simulink model "Estim_DistCont_Fault_topresent"  (R2018b)
settings: Solver=ode1  StartTime=0.0  StopTime=20000  FixedStep=1  RelTol=1e-3
InitFcn:
  | clearvars
  | addpath('C:\Users\u375749\Documents\Thesis\Codes\Linearization')
  | addpath('C:\Users\u375749\Documents\Thesis\Codes\MatlabPlant')
  | addpath('C:\Users\u375749\Documents\Thesis\Codes\ModelicaPlant\objects_inits')
  | addpath('C:\Users\u375749\Documents\Thesis\Codes\ModelicaPlant\matfiles')
  | addpath('C:\Users\u375749\Documents\Thesis\Codes\ModelicaPlant')
  | modelcreation_simplified
  | substitution_simplified
  | distributedControllers
  | delayT = 300;
  | delayh = 50;% 400*19.2*1e-3*2/0.321;
  | hRatio = 1/3;
  | kfinit_simulink
  | rlsinit_simulink
  | enableFaultOperation = 1;
  | enableBatch = 0;
  | enableTA0fault = 0;
  | faultinit_simulink
  | clear u
values from neighbouring files (symbols this model uses):
  fValues = 48    [faultcontrol3.mat]    (also in faultcontrol4.mat)
  npy = 2    [faultcontrol3.mat]    (also in faultcontrol4.mat)
  nr = 6    [faultcontrol3.mat]    (also in faultcontrol4.mat)
  sigma2p = 277777777.778    [faultcontrol3.mat]    (also in faultcontrol4.mat)
  sigma2T = 0.111111111111    [faultcontrol3.mat]    (also in faultcontrol4.mat)
  sigma2x = 1.11111111111e-05    [faultcontrol3.mat]    (also in faultcontrol4.mat)
  Ts = 1    [faultcontrol3.mat]    (also in faultcontrol4.mat)
  VValues = [0.0192 0.133 0.0001 0.00024]    [faultcontrol3.mat]    (also in faultcontrol4.mat)
undefined symbols (not defined in the file or in its folder): CoolProp, DiscIntNeverNeededParam, fdEM, PI_C, PI_F, PI_GC, PI_HP, PI_LT, PI_MT, PI_RP, rls, x2q
libraries: simulink x6, dspswit3 x1, FMIKit_blocks x1
settings Model: NumberOfSteps=10  Creator=U370698  LastModifiedBy=U375749
settings DebuggingCC: LibraryContextMissingDiagnostic=none  UnderSpecifiedDimensionMsg=warning
settings SFSimCC: SimUseLocalCustomCode=off
settings RTWCC: RTWUseLocalCustomCode=off

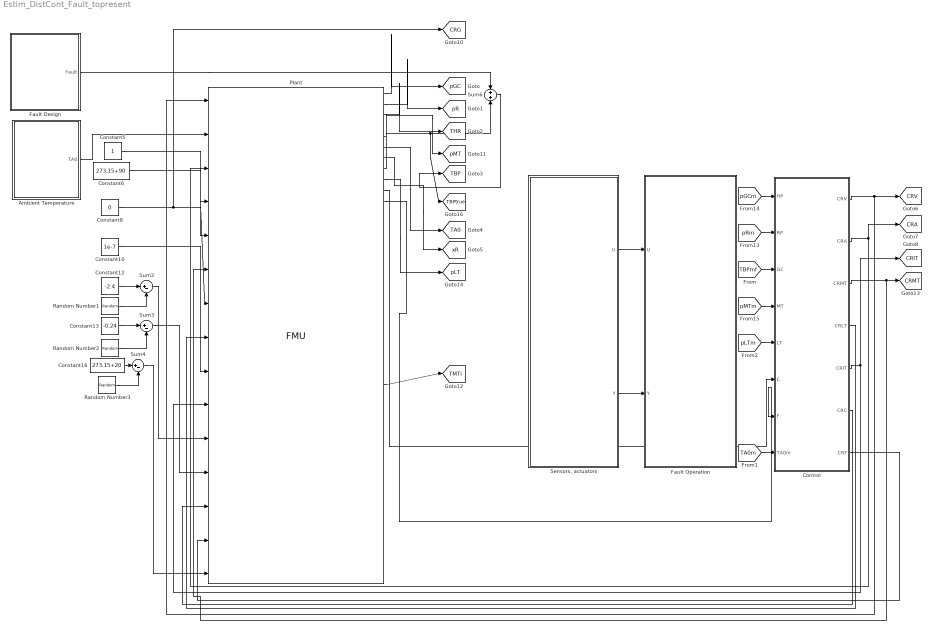
== system Estim_DistCont_Fault_topresent ==
  Ambient Temperature : Subsystem
  Constant10 : Constant  Value=1e-7
  Constant12 : Constant  Value=-2.4
  Constant13 : Constant  Value=-0.24
  Constant16 : Constant  Value=273.15+20
  Constant5 : Constant
  Constant6 : Constant  Value=273.15+90
  Constant8 : Constant  Value=0
  Control : Subsystem
  Fault Design : Subsystem
  Fault Operation : Subsystem
  Plant : FMIKit_blocks/FMU  SFunctionModules=''
      settings: SourceProductName=FMI Kit
  Random Number1 : RandomNumber  Variance=(0.2/3)^2/Ts  Seed=51  SampleTime=1
  Random Number2 : RandomNumber  Variance=(0.02/3)^2/Ts  Seed=52  SampleTime=1
  Random Number3 : RandomNumber  Variance=(1/10)^2/Ts  Seed=53  SampleTime=1
  "Sensors, actuators" : Subsystem
  Sum2 : Sum  Inputs=|+-
  Sum3 : Sum  Inputs=|+-
  Sum4 : Sum  Inputs=|+-
  Sum6 : Sum  Inputs=+|+
  tag scope: CRA=global, CRG=global, CRIT=global, CRMT=global, CRV=global, TA0=global, TBP=global, TBPtrue=global, THR=global, TMTi=global, pGC=global, pLT=global, pMT=global, pR=global, xR=global
  wires:
  Constant5/1 -> Plant/4
  Constant6/1 -> Plant/5
  Constant8/1 -> [CRG], Plant/7
  Constant10/1 -> Plant/9
  Plant/1 -> [pGC]
  Plant/3 -> [THR]
  Control/1(CRV) -> [CRV], Plant/1
  Control/2(CRA) -> [CRA], Plant/3
  Control/3(CRMT) -> Plant/6, [CRMT]
  Control/4(CRLT) -> Plant/8
  Control/6(CRC) -> Plant/13
  Control/7(CRF) -> Plant/14
  Plant/11 -> Control/7(F)
  Plant/10 -> Control/6(C)
  Plant/9 -> [pLT]
  Plant/8 -> [pMT]
  Plant/7 -> [xR]
  Plant/6 -> [TA0]
  Sum6/1 -> [TBP]
  Plant/2 -> [pR]
  Control/5(CRIT) -> [CRIT], Plant/10
  "Sensors, actuators"/1(U) -> Fault Operation/1(U)
  "Sensors, actuators"/2(Y) -> Fault Operation/2(Y)
  Constant12/1 -> Sum2/1
  Sum2/1 -> Plant/11
  Constant13/1 -> Sum3/1
  Sum3/1 -> Plant/12
  Random Number1/1 -> Sum2/2
  Random Number2/1 -> Sum3/2
  Constant16/1 -> Sum4/1
  Sum4/1 -> Plant/15
  Random Number3/1 -> Sum4/2
  Plant/5 -> [TBPtrue], Sum6/2
  Plant/28 -> [TMTi]
  [pGCm] -> Control/1(HP)
  [pRm] -> Control/2(RP)
  [TBPmf] -> Control/3(GC)
  [pLTm] -> Control/5(LT)
  [pMTm] -> Control/4(MT)
  Fault Design/1(Fault) -> Sum6/1
  [TA0m] -> Control/8(TA0m)
  Ambient Temperature/1(TA0) -> Plant/2

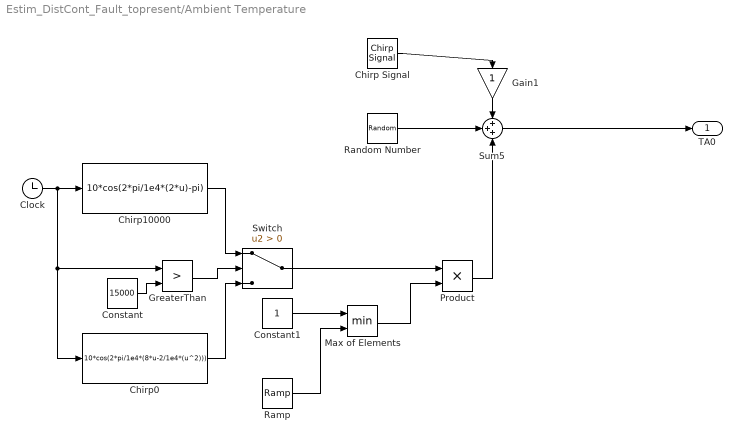
== system Estim_DistCont_Fault_topresent/Ambient Temperature ==
  Chirp Signal : simulink/Sources/Chirp Signal  f1=2*pi/10000  T=10000  f2=2*pi*10/10000
  Chirp0 : MATLABFcn  MATLABFcn=10*cos(2*pi/1e4*(8*u-2/1e4*(u^2)))  OutputDimensions=1
  Chirp10000 : MATLABFcn  MATLABFcn=10*cos(2*pi/1e4*(2*u)-pi)  OutputDimensions=1
  Clock : Clock
  Constant : Constant  Value=15000
  Constant1 : Constant
  Gain1 : Gain
  GreaterThan : RelationalOperator  Operator=>  OutDataTypeStr=boolean  RndMeth=Simplest
  Max of Elements : MinMax  Inputs=2
  Product : Product
  Ramp : simulink/Sources/Ramp  slope=0.75/(10000-6000)  start=6000  InitialOutput=0.25
  Random Number : RandomNumber  Mean=273.15+20  Variance=(1/10)^2/Ts  Seed=50  SampleTime=1
  Sum5 : Sum  Inputs=+++
  Switch : Switch  Criteria=u2 > Threshold
  TA0 : Outport
  wires:
  Random Number/1 -> Sum5/2
  Gain1/1 -> Sum5/1
  Sum5/1 -> TA0/1
  Chirp Signal/1 -> Gain1/1
  Product/1 -> Sum5/3
  Max of Elements/1 -> Product/2
  Ramp/1 -> Max of Elements/2
  Chirp10000/1 -> Switch/1
  Constant/1 -> GreaterThan/2
  Switch/1 -> Product/1
  GreaterThan/1 -> Switch/2
  Chirp0/1 -> Switch/3
  Constant1/1 -> Max of Elements/1
  Clock/1 -> Chirp0/1, GreaterThan/1, Chirp10000/1

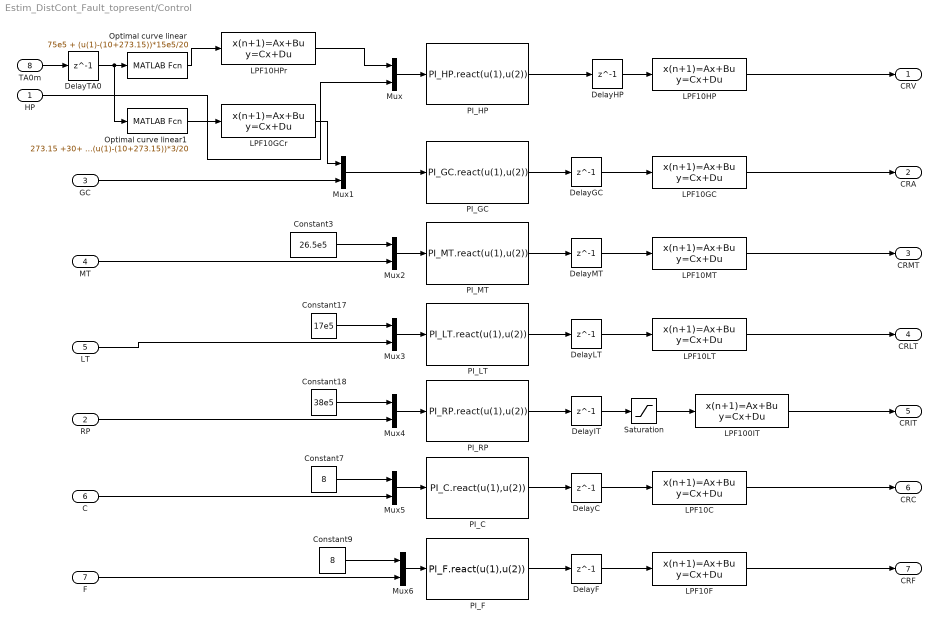
== system Estim_DistCont_Fault_topresent/Control ==
  HP : Inport
  RP : Inport  Port=2
  GC : Inport  Port=3
  MT : Inport  Port=4
  LT : Inport  Port=5
  C : Inport  Port=6
  F : Inport  Port=7
  TA0m : Inport  Port=8
  Constant17 : Constant  Value=17e5
  Constant18 : Constant  Value=38e5
  Constant3 : Constant  Value=26.5e5
  Constant7 : Constant  Value=8
  Constant9 : Constant  Value=8
  DelayC : Delay  DelayLength=1  InitialCondition=0.1
  DelayF : Delay  DelayLength=1  InitialCondition=0.04
  DelayGC : Delay  DelayLength=1  InitialCondition=0.625
  DelayHP : Delay  DelayLength=1  InitialCondition=0.25
  DelayIT : Delay  DelayLength=1  InitialCondition=0.45
  DelayLT : Delay  DelayLength=1  InitialCondition=0.3
  DelayMT : Delay  DelayLength=1  InitialCondition=0.3
  DelayTA0 : Delay  DelayLength=1  InitialCondition=273.15+30
  LPF100IT : DiscreteStateSpace  A=0.99  B=0.125  C=0.0796  D=0  InitialCondition=0.45  SampleTime=-1
  LPF10C : DiscreteStateSpace  A=0.9048  B=0.25  C=0.3807  D=0  InitialCondition=0.1  SampleTime=-1
  LPF10F : DiscreteStateSpace  A=0.9048  B=0.25  C=0.3807  D=0  InitialCondition=0.04  SampleTime=-1
  LPF10GC : DiscreteStateSpace  A=0.9048  B=0.25  C=0.3807  D=0  InitialCondition=0.625  SampleTime=-1
  LPF10GCr : DiscreteStateSpace  A=0.9048  B=0.25  C=0.3807  D=0  InitialCondition=273.15+33  SampleTime=-1
  LPF10HP : DiscreteStateSpace  A=0.9048  B=0.25  C=0.3807  D=0  InitialCondition=0.25  SampleTime=-1
  LPF10HPr : DiscreteStateSpace  A=0.9048  B=0.25  C=0.3807  D=0  InitialCondition=85e5  SampleTime=-1
  LPF10LT : DiscreteStateSpace  A=0.9048  B=0.25  C=0.3807  D=0  InitialCondition=0.3  SampleTime=-1
  LPF10MT : DiscreteStateSpace  A=0.9048  B=0.25  C=0.3807  D=0  InitialCondition=0.3  SampleTime=-1
  Mux{,1..6} (7 alike) : Mux  Inputs=2
  Optimal curve linear : MATLABFcn  MATLABFcn=75e5 + (u(1)-(10+273.15))*15e5/20
  Optimal curve linear1 : MATLABFcn  MATLABFcn=273.15 +30+ (u(1)-(10+273.15))*3/20
  PI_C : MATLABFcn  MATLABFcn=PI_C.react(u(1),u(2))
  PI_F : MATLABFcn  MATLABFcn=PI_F.react(u(1),u(2))
  PI_GC : MATLABFcn  MATLABFcn=PI_GC.react(u(1),u(2))
  PI_HP : MATLABFcn  MATLABFcn=PI_HP.react(u(1),u(2))
  PI_LT : MATLABFcn  MATLABFcn=PI_LT.react(u(1),u(2))
  PI_MT : MATLABFcn  MATLABFcn=PI_MT.react(u(1),u(2))
  PI_RP : MATLABFcn  MATLABFcn=PI_RP.react(u(1),u(2))
  Saturation : Saturate  UpperLimit=0.7  LowerLimit=0
  CRV : Outport
  CRA : Outport  Port=2
  CRMT : Outport  Port=3
  CRLT : Outport  Port=4
  CRIT : Outport  Port=5
  CRC : Outport  Port=6
  CRF : Outport  Port=7
  wires:
  MT/1 -> Mux2/2
  Mux3/1 -> PI_LT/1
  Mux4/1 -> PI_RP/1
  DelayHP/1 -> LPF10HP/1
  DelayLT/1 -> LPF10LT/1
  LPF10GCr/1 -> Mux1/1
  Mux6/1 -> PI_F/1
  PI_HP/1 -> DelayHP/1
  Optimal curve linear/1 -> LPF10HPr/1
  PI_MT/1 -> DelayMT/1
  PI_LT/1 -> DelayLT/1
  PI_GC/1 -> DelayGC/1
  Mux2/1 -> PI_MT/1
  Constant18/1 -> Mux4/1
  Mux5/1 -> PI_C/1
  Constant7/1 -> Mux5/1
  Constant3/1 -> Mux2/1
  Constant9/1 -> Mux6/1
  PI_C/1 -> DelayC/1
  PI_F/1 -> DelayF/1
  PI_RP/1 -> DelayIT/1
  F/1 -> Mux6/2
  HP/1 -> Mux/2
  Constant17/1 -> Mux3/1
  Mux/1 -> PI_HP/1
  GC/1 -> Mux1/2
  LT/1 -> Mux3/2
  DelayC/1 -> LPF10C/1
  DelayF/1 -> LPF10F/1
  C/1 -> Mux5/2
  DelayGC/1 -> LPF10GC/1
  DelayMT/1 -> LPF10MT/1
  RP/1 -> Mux4/2
  LPF10HP/1 -> CRV/1
  LPF10GC/1 -> CRA/1
  LPF10MT/1 -> CRMT/1
  LPF10LT/1 -> CRLT/1
  LPF100IT/1 -> CRIT/1
  LPF10C/1 -> CRC/1
  LPF10F/1 -> CRF/1
  DelayIT/1 -> Saturation/1
  Saturation/1 -> LPF100IT/1
  LPF10HPr/1 -> Mux/1
  Optimal curve linear1/1 -> LPF10GCr/1
  TA0m/1 -> DelayTA0/1
  DelayTA0/1 -> Optimal curve linear1/1, Optimal curve linear/1
  Mux1/1 -> PI_GC/1

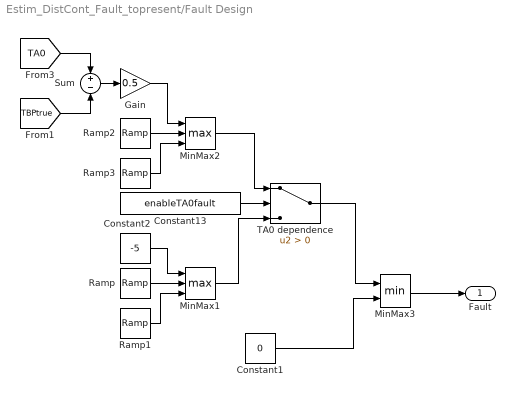
== system Estim_DistCont_Fault_topresent/Fault Design ==
  Constant1 : Constant  Value=0
  Constant13 : Constant  Value=enableTA0fault
  Constant2 : Constant  Value=-5
  Gain : Gain  Gain=0.5
  MinMax1 : MinMax  Function=max  Inputs=3
  MinMax2 : MinMax  Function=max  Inputs=3
  MinMax3 : MinMax  Inputs=2
  Ramp : simulink/Sources/Ramp  slope=-1/10  start=5000  InitialOutput=0
  Ramp1 : simulink/Sources/Ramp  slope=1/10  start=12000  InitialOutput=-5
  Ramp2 : simulink/Sources/Ramp  slope=-1/100  start=5000  InitialOutput=0
  Ramp3 : simulink/Sources/Ramp  slope=1/100  start=12000  InitialOutput=-20
  Sum : Sum  Inputs=+|-
  TA0 dependence : Switch  Criteria=u2 > Threshold
  Fault : Outport
  wires:
  Ramp/1 -> MinMax1/2
  Constant1/1 -> MinMax3/2
  MinMax3/1 -> Fault/1
  Ramp1/1 -> MinMax1/3
  Constant13/1 -> TA0 dependence/2
  Sum/1 -> Gain/1
  [TA0] -> Sum/1
  [TBPtrue] -> Sum/2
  Constant2/1 -> MinMax1/1
  MinMax1/1 -> TA0 dependence/3
  Gain/1 -> MinMax2/1
  Ramp3/1 -> MinMax2/3
  Ramp2/1 -> MinMax2/2
  TA0 dependence/1 -> MinMax3/1
  MinMax2/1 -> TA0 dependence/1

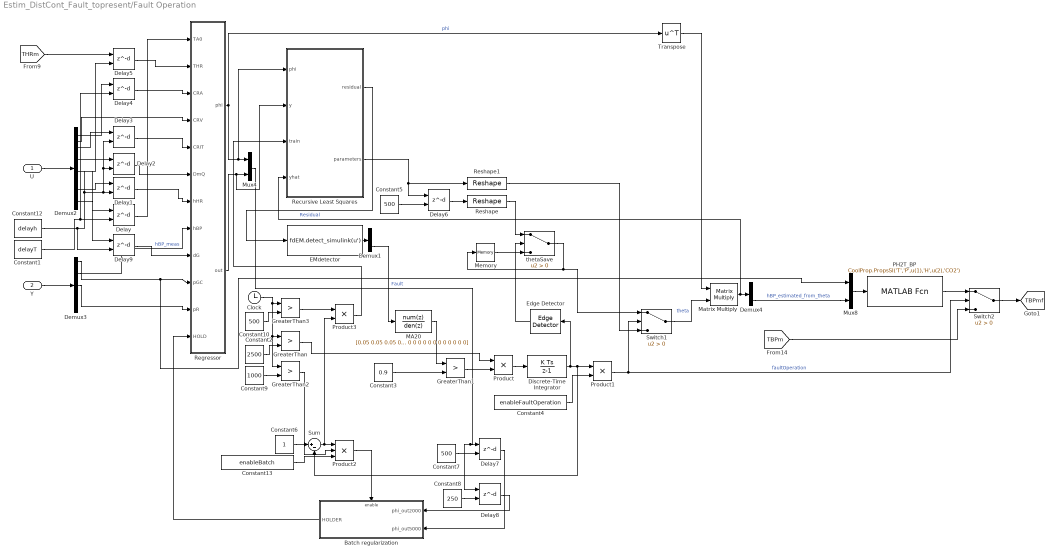
== system Estim_DistCont_Fault_topresent/Fault Operation ==
  U : Inport
  Y : Inport  Port=2
  Batch regularization : Subsystem
  Clock : Clock
  Constant1 : Constant  Value=delayT
  Constant10 : Constant  Value=500
  Constant12 : Constant  Value=delayh
  Constant13 : Constant  Value=enableBatch
  Constant2 : Constant  Value=2500
  Constant3 : Constant  Value=0.9
  Constant4 : Constant  Value=enableFaultOperation
  Constant5 : Constant  Value=500
  Constant6 : Constant
  Constant7 : Constant  Value=500
  Constant8 : Constant  Value=250
  Constant9 : Constant  Value=1000
  Delay : Delay  DelayLengthSource=Input port  DelayLength=delayh  DelayLengthUpperLimit=1000  InitialCondition=30+273
      settings: InputPortMap=u0,p1
  Delay1 : Delay  DelayLengthSource=Input port  DelayLength=delayh  DelayLengthUpperLimit=1000  InitialCondition=525e3
      settings: InputPortMap=u0,p1
  Delay2 : Delay  DelayLengthSource=Input port  DelayLength=delayh  DelayLengthUpperLimit=1000  InitialCondition=0.5
      settings: InputPortMap=u0,p1
  Delay3 : Delay  DelayLengthSource=Input port  DelayLength=delayh  DelayLengthUpperLimit=1000  InitialCondition=0.5
      settings: InputPortMap=u0,p1
  Delay4 : Delay  DelayLengthSource=Input port  DelayLength=delayh  DelayLengthUpperLimit=1000  InitialCondition=0.5
      settings: InputPortMap=u0,p1
  Delay5 : Delay  DelayLengthSource=Input port  DelayLength=delayh  DelayLengthUpperLimit=1000  InitialCondition=30+273
      settings: InputPortMap=u0,p1
  Delay6 : Delay  DelayLengthSource=Input port  DelayLength=delayh  DelayLengthUpperLimit=500  InitialCondition=zeros(size(rls.t,1)*size(rls.t,2),500)
      settings: InputPortMap=u0,p1
  Delay7 : Delay  DelayLengthSource=Input port  DelayLength=delayh  DelayLengthUpperLimit=500  InitialCondition=zeros(size(rls.t,1)+size(rls.t,2),500)
      settings: InputPortMap=u0,p1
  Delay8 : Delay  DelayLengthSource=Input port  DelayLength=delayh  DelayLengthUpperLimit=250  InitialCondition=zeros(size(rls.t,1)+size(rls.t,2),250)
      settings: InputPortMap=u0,p1
  Delay9 : Delay  DelayLengthSource=Input port  DelayLength=delayh  DelayLengthUpperLimit=1000  InitialCondition=80
      settings: InputPortMap=u0,p1
  Demux1 : Demux  Outputs=[1 1]
  Demux2 : Demux  Outputs=12
  Demux3 : Demux  Outputs=5
  Demux4 : Demux  Outputs=2
  Discrete-Time Integrator : DiscreteIntegrator  SampleTime=-1  LimitOutput=on  UpperSaturationLimit=1  LowerSaturationLimit=0  ICPrevOutput=DiscIntNeverNeededParam  ICPrevScaledInput=DiscIntNeverNeededParam
  EMdetector : MATLABFcn  MATLABFcn=fdEM.detect_simulink(u')  OutputDimensions=2
  Edge Detector : dspswit3/Edge Detector  InputProcessing=Columns as channels (frame based)
      settings: SourceProductName=DSP System Toolbox  SourceProductBaseCode=DS
  GreaterThan{,1..3} (4 alike) : RelationalOperator  Operator=>  OutDataTypeStr=boolean  RndMeth=Simplest
  MA20 : DiscreteTransferFcn  Numerator=[0.05 0.05 0.05 0.05 0.05 0.05 0.05 0.05 0.05 0.05 0.05 0.05 0.05 0.05 0.05 0.05 0.05 0.05 0.05 0.05]  Denominator=[1 0 0 0 0 0 0 0 0 0 0 0 0 0 0 0 0 0 0 0]  InitialStates=zeros(1,19)  a0EqualsOne=on
  Matrix Multiply : Product  Multiplication=Matrix(*)
  Memory : Memory  InitialCondition=zeros(size(rls.t,1),size(rls.t,2))  InheritSampleTime=on  LinearizeAsDelay=on
  Mux4 : Mux  Inputs=[size(rls.t,1) size(rls.t,2)]
  Mux8 : Mux  Inputs=2
  PH2T_BP : MATLABFcn  MATLABFcn=CoolProp.PropsSI('T','P',u(1),'H',u(2),'CO2')  OutputDimensions=1
  Product : Product
  Product1 : Product
  Product2 : Product  Inputs=3
  Product3 : Product
  Recursive Least Squares : Subsystem
  Regressor : MATLAB Function  TreatAsAtomicUnit=on
  Reshape : Reshape  OutputDimensionality=Customize  OutputDimensions=[size(rls.t,1),size(rls.t,2)]
  Reshape1 : Reshape  OutputDimensionality=Customize  OutputDimensions=[size(rls.t,1),size(rls.t,2)]
  Sum : Sum  Inputs=|+-
  Switch1 : Switch  Criteria=u2 > Threshold
  Switch2 : Switch  Criteria=u2 > Threshold
  Transpose : Math  Operator=transpose  SaturateOnIntegerOverflow=on
  thetaSave : Switch  Criteria=u2 > Threshold
  tag scope: TBPmf=global
  wires:
  Y/1 -> Demux3/1
  U/1 -> Demux2/1
  Mux4/1 -> Delay8/1, Delay7/1
  Regressor/2(out) -> Recursive Least Squares/2(y), Mux4/2
  Regressor/1(phi) -> Recursive Least Squares/1(phi), Mux4/1, Transpose/1  "phi"
  Constant1/1 -> Delay4/2, Delay/2
  Demux2/12 -> Delay/1
  Delay/1 -> Regressor/1(TA0)
  Demux3/1 -> Mux8/1, Regressor/10(pGC)
  Demux2/10 -> Delay1/1
  Constant12/1 -> Delay9/2, Delay5/2, Delay3/2, Delay2/2, Delay1/2
  Demux2/3 -> Delay3/1
  Delay3/1 -> Regressor/5(CRIT)
  Demux2/1 -> Delay4/1
  Delay4/1 -> Regressor/3(CRA)
  Demux3/3 -> Regressor/11(pR)
  Demux3/2 -> Regressor/8(hBP)  "hBP_meas"
  Delay1/1 -> Regressor/7(hHR)
  Demux2/5 -> Delay2/1
  Delay2/1 -> Regressor/6(DmQ)
  [THRm] -> Delay5/1
  Delay5/1 -> Regressor/2(THR)
  Clock/1 -> GreaterThan2/1, GreaterThan/1, GreaterThan3/1
  Constant2/1 -> GreaterThan/2
  Recursive Least Squares/2(parameters) -> Delay6/1, Reshape1/1
  Constant3/1 -> GreaterThan1/2
  Recursive Least Squares/1(residual) -> EMdetector/1  "Residual"
  EMdetector/1 -> Demux1/1
  Demux1/2 -> MA20/1  "Fault"
  Transpose/1 -> Matrix Multiply/1
  Delay6/1 -> Reshape/1
  GreaterThan1/1 -> Product/2
  GreaterThan/1 -> Product/1
  Product/1 -> Discrete-Time Integrator/1
  Memory/1 -> thetaSave/3
  Edge Detector/1 -> thetaSave/2
  thetaSave/1 -> Memory/1, Switch1/1
  Product1/1 -> Switch2/2, Switch1/2  "faultOperation"
  Switch1/1 -> Matrix Multiply/2  "theta"
  Matrix Multiply/1 -> Recursive Least Squares/4(yhat), Demux4/1
  Constant4/1 -> Product1/2
  Demux2/2 -> Regressor/4(CRV)
  Mux8/1 -> PH2T_BP/1
  PH2T_BP/1 -> Switch2/1
  Switch2/1 -> [TBPmf]
  Demux4/2 -> Mux8/2  "hBP_estimated_from_theta"
  Constant5/1 -> Delay6/2
  Discrete-Time Integrator/1 -> Product1/1, Sum/2, Edge Detector/1
  MA20/1 -> GreaterThan1/1
  Reshape/1 -> thetaSave/1
  Reshape1/1 -> Switch1/3
  Sum/1 -> Product2/1, Product3/2
  Constant6/1 -> Sum/1
  Batch regularization/1(HOLDER) -> Regressor/12(HOLD)
  Constant7/1 -> Delay7/2
  Constant8/1 -> Delay8/2
  Delay8/1 -> Batch regularization/1(phi_out2000)
  Delay7/1 -> Batch regularization/2(phi_out5000)
  Constant9/1 -> GreaterThan2/2
  GreaterThan2/1 -> Product2/2
  Demux2/7 -> Delay9/1
  Delay9/1 -> Regressor/9(dG)
  Constant10/1 -> GreaterThan3/2
  [TBPm] -> Switch2/3
  Product2/1 -> Batch regularization/Enable
  GreaterThan3/1 -> Product3/1
  Product3/1 -> Recursive Least Squares/3(train)
  Constant13/1 -> Product2/3

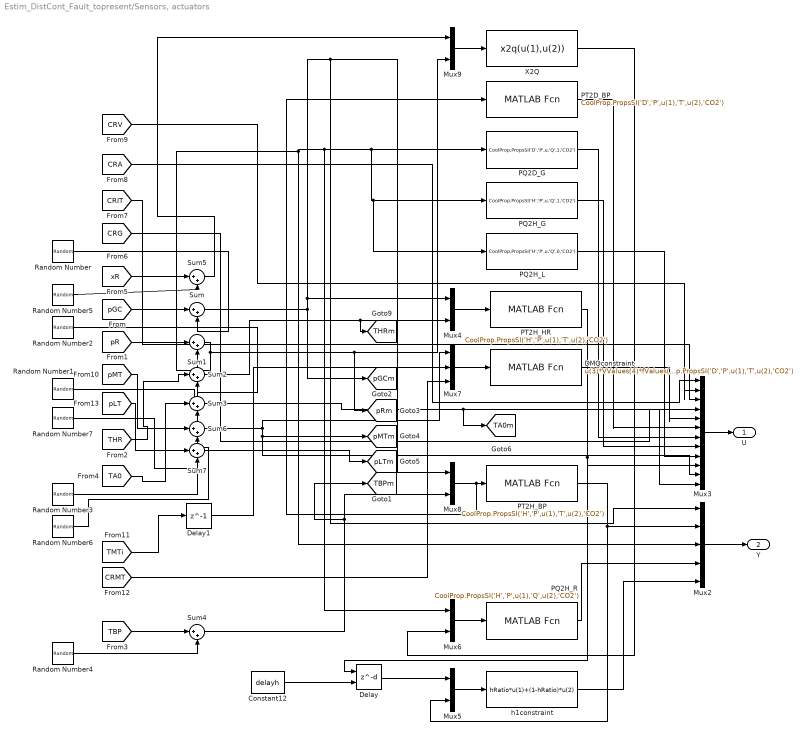
== system Estim_DistCont_Fault_topresent/Sensors, actuators ==
  Constant12 : Constant  Value=delayh
  DMQconstraint : MATLABFcn  MATLABFcn=u(3)*VValues(4)*fValues(1)*CoolProp.PropsSI('D','P',u(1),'T',u(2),'CO2')
  Delay : Delay  DelayLengthSource=Input port  DelayLength=delayh  DelayLengthUpperLimit=1000  InitialCondition=525e3
      settings: InputPortMap=u0,p1
  Delay1 : Delay  DelayLength=1  InitialCondition=270
  Mux2 : Mux  Inputs=5
  Mux3 : Mux  Inputs=12
  Mux{4..6,8..9} (5 alike) : Mux  Inputs=2
  Mux7 : Mux  Inputs=3
  PQ2D_G : MATLABFcn  MATLABFcn=CoolProp.PropsSI('D','P',u,'Q',1,'CO2')
  PQ2H_G : MATLABFcn  MATLABFcn=CoolProp.PropsSI('H','P',u,'Q',1,'CO2')
  PQ2H_L : MATLABFcn  MATLABFcn=CoolProp.PropsSI('H','P',u,'Q',0,'CO2')
  PQ2H_R : MATLABFcn  MATLABFcn=CoolProp.PropsSI('H','P',u(1),'Q',u(2),'CO2')
  PT2D_BP : MATLABFcn  MATLABFcn=CoolProp.PropsSI('D','P',u(1),'T',u(2),'CO2')
  PT2H_BP : MATLABFcn  MATLABFcn=CoolProp.PropsSI('H','P',u(1),'T',u(2),'CO2')  OutputDimensions=1
  PT2H_HR : MATLABFcn  MATLABFcn=CoolProp.PropsSI('H','P',u(1),'T',u(2),'CO2')
  Random Number : RandomNumber  Variance=sigma2p/Ts  SampleTime=1
  Random Number1 : RandomNumber  Variance=sigma2T/Ts  Seed=10  SampleTime=1
  Random Number2 : RandomNumber  Variance=sigma2p/Ts  Seed=1  SampleTime=1
  Random Number3 : RandomNumber  Variance=sigma2T/Ts  Seed=12  SampleTime=1
  Random Number4 : RandomNumber  Variance=sigma2T/Ts  Seed=11  SampleTime=1
  Random Number5 : RandomNumber  Variance=sigma2x/Ts  Seed=21  SampleTime=1
  Random Number6 : RandomNumber  Variance=sigma2p/Ts  Seed=111  SampleTime=1
  Random Number7 : RandomNumber  Variance=sigma2T/Ts  Seed=10  SampleTime=112
  Sum{,1..7} (8 alike) : Sum  Inputs=|++
  X2Q : MATLABFcn  MATLABFcn=x2q(u(1),u(2))
  h1constraint : MATLABFcn  MATLABFcn=hRatio*u(1)+(1-hRatio)*u(2)
  U : Outport
  Y : Outport  Port=2
  tag scope: TA0m=global, TBPm=global, THRm=global, pGCm=global, pLTm=global, pMTm=global, pRm=global
  wires:
  Sum1/1 -> Mux6/1, PQ2H_L/1, PQ2H_G/1, PQ2D_G/1, Mux2/3, [pRm], Mux9/2
  PT2H_HR/1 -> Delay/1, Mux3/10
  Sum/1 -> [pGCm], Mux2/1, Mux8/1, Mux4/1
  PQ2H_L/1 -> Mux3/9
  Sum5/1 -> Mux9/1
  [CRIT] -> Mux3/3
  PQ2H_R/1 -> Mux2/4
  PT2D_BP/1 -> Mux3/6
  DMQconstraint/1 -> Mux3/5
  Mux9/1 -> X2Q/1
  [CRV] -> Mux3/2
  [CRA] -> Mux3/1
  PT2H_BP/1 -> Mux5/2, Mux2/2
  PQ2D_G/1 -> Mux3/7
  Mux8/1 -> PT2D_BP/1, PT2H_BP/1
  Mux4/1 -> PT2H_HR/1
  X2Q/1 -> Mux6/2
  PQ2H_G/1 -> Mux3/8
  Mux6/1 -> PQ2H_R/1
  Mux3/1 -> U/1
  Mux2/1 -> Y/1
  [pGC] -> Sum/1
  Random Number/1 -> Sum/2
  [pR] -> Sum1/1
  Random Number2/1 -> Sum1/2
  Sum2/1 -> [THRm], Mux4/2
  [THR] -> Sum2/1
  Random Number1/1 -> Sum2/2
  [TA0] -> Sum3/1
  Random Number3/1 -> Sum3/2
  [TBP] -> Sum4/1
  Random Number4/1 -> Sum4/2
  Random Number5/1 -> Sum5/2
  [xR] -> Sum5/1
  Mux5/1 -> h1constraint/1
  Sum4/1 -> Mux8/2, [TBPm]
  Delay/1 -> Mux5/1
  h1constraint/1 -> Mux2/5
  Sum3/1 -> [TA0m], Mux3/12
  [CRG] -> Mux3/4
  Sum6/1 -> Mux3/11, [pMTm], Mux7/1
  Mux7/1 -> DMQconstraint/1
  [CRMT] -> Mux7/3
  [TMTi] -> Delay1/1
  Delay1/1 -> Mux7/2
  Constant12/1 -> Delay/2
  Random Number6/1 -> Sum6/2
  [pMT] -> Sum6/1
  Random Number7/1 -> Sum7/2
  [pLT] -> Sum7/1
  Sum7/1 -> [pLTm]

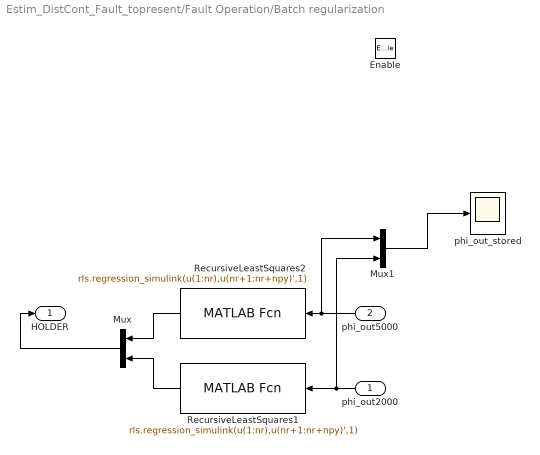
== system Estim_DistCont_Fault_topresent/Fault Operation/Batch regularization ==
  phi_out2000 : Inport
  phi_out5000 : Inport  Port=2
  Enable : EnablePort
  Mux : Mux  Inputs=2
  Mux1 : Mux  Inputs=2
  RecursiveLeastSquares1 : MATLABFcn  MATLABFcn=rls.regression_simulink(u(1:nr),u(nr+1:nr+npy)',1)  OutputDimensions=length(rls.e)+size(rls.t,1)*size(rls.t,2)  Output1D=off
  RecursiveLeastSquares2 : MATLABFcn  MATLABFcn=rls.regression_simulink(u(1:nr),u(nr+1:nr+npy)',1)  OutputDimensions=length(rls.e)+size(rls.t,1)*size(rls.t,2)  Output1D=off
  phi_out_stored : Scope
  HOLDER : Outport
  wires:
  phi_out2000/1 -> Mux1/2, RecursiveLeastSquares1/1
  Mux/1 -> HOLDER/1
  RecursiveLeastSquares2/1 -> Mux/1
  RecursiveLeastSquares1/1 -> Mux/2
  phi_out5000/1 -> Mux1/1, RecursiveLeastSquares2/1
  Mux1/1 -> phi_out_stored/1

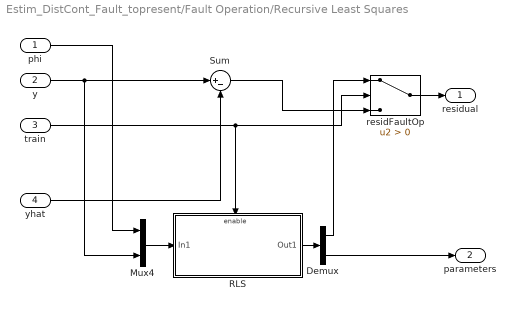
== system Estim_DistCont_Fault_topresent/Fault Operation/Recursive Least Squares ==
  phi : Inport
  y : Inport  Port=2
  train : Inport  Port=3
  yhat : Inport  Port=4
  Demux : Demux  Outputs=[length(rls.e) size(rls.t,1)*size(rls.t,2)]
  Mux4 : Mux  Inputs=[size(rls.t,1) size(rls.t,2)]
  RLS : Subsystem
  Sum : Sum  Inputs=|+-
  residFaultOp : Switch  Criteria=u2 > Threshold
  residual : Outport
  parameters : Outport  Port=2
  wires:
  train/1 -> residFaultOp/2, RLS/Enable
  residFaultOp/1 -> residual/1
  Demux/2 -> parameters/1
  Mux4/1 -> RLS/1(In1)
  RLS/1(Out1) -> Demux/1
  y/1 -> Sum/1, Mux4/2
  phi/1 -> Mux4/1
  yhat/1 -> Sum/2
  Demux/1 -> residFaultOp/1
  Sum/1 -> residFaultOp/3

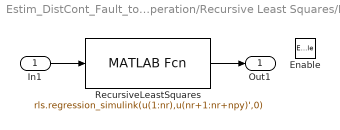
== system Estim_DistCont_Fault_topresent/Fault Operation/Recursive Least Squares/RLS ==
  In1 : Inport
  Enable : EnablePort
  RecursiveLeastSquares : MATLABFcn  MATLABFcn=rls.regression_simulink(u(1:nr),u(nr+1:nr+npy)',0)  OutputDimensions=length(rls.e)+size(rls.t,1)*size(rls.t,2)  Output1D=off
  Out1 : Outport
  wires:
  In1/1 -> RecursiveLeastSquares/1
  RecursiveLeastSquares/1 -> Out1/1

== matlab function Estim_DistCont_Fault_topresent/Fault Operation/Regressor ==
  data: TA0 input; phi output; THR input; out output; CRA input; CRV input; CRIT input; DmQ input; hHR input; hBP input; dG input; pGC input; pR input; HOLD input
function [phi,out] = fcn(TA0,THR,CRA,CRV,CRIT,DmQ,hHR,hBP,dG,pGC,pR,HOLD)

% DmV = CRV*0.8*3e-5*sqrt(dBP*(pGC - pR));
DmIT = dG*1e-4*CRIT*48;
DmV = DmQ + DmIT;
DQ = DmV*(hHR - hBP);
% phi = [1; hHR; TA0; (THR-TA0); CRA; CRIT*hHR; DmQ*hHR; CRV*sqrt(pGC-pR)];
phi = [1; hHR; (THR-TA0); CRA; DmIT*hHR; DmQ*hHR; CRV*sqrt(pGC-pR)];
out = [DQ hBP]';
